simulink model "robot_joint_controlled_3_state"  (R2017b)
settings: Solver=ode8  StartTime=0.0  StopTime=2.0  FixedStep=0.00001  RelTol=1e-3
model workspace: external: MATLAB File D:\Projects\SERTS\Body\v7.0\Matlab\robot_DataFile.m (data not in the file)
values from neighbouring files (symbols this model uses):
  c_roll = 60    [best_so_far_variables.m]    (also in variables.m = 50)
  c_stance = [30,   0,    0 ... (first row only)    [best_so_far_variables.m]    (also in variables.m)
  c_swing = [50,   0,    0 ... (first row only)    [best_so_far_variables.m]    (also in variables.m = [100,   0,    0)
  c_yaw = 60    [best_so_far_variables.m]    (also in variables.m = 30)
  desired_body_height = 0.6    [best_so_far_variables.m]    (also in variables.m)
  desired_body_x_velocity = 0    [best_so_far_variables.m]    (also in variables.m)
  desired_body_y_velocity = 1    [best_so_far_variables.m]    (also in variables.m)
  desired_yaw = 0    [best_so_far_variables.m]    (also in variables.m)
  k_roll = 300    [best_so_far_variables.m]    (also in variables.m = 700)
  k_stance = [    0,    0,       0 ... (first row only)    [best_so_far_variables.m]    (also in variables.m)
  k_swing = [ 1000,     0,       0 ... (first row only)    [best_so_far_variables.m]    (also in variables.m = [02000,     0,       0)
  k_x = 0.03    [best_so_far_variables.m]    (also in variables.m)
  k_y = 0.03    [best_so_far_variables.m]    (also in variables.m)
  k_yaw = 300    [best_so_far_variables.m]    (also in variables.m)
  Left = 1    [best_so_far_variables.m]    (also in variables.m)
  LF_RH = -1    [best_so_far_variables.m]    (also in variables.m)
  lift_height = 0.05    [best_so_far_variables.m]    (also in variables.m)
  RF_LH = 1    [best_so_far_variables.m]    (also in variables.m)
  Right = -1    [best_so_far_variables.m]    (also in variables.m)
  stance_time = 0.2    [best_so_far_variables.m]    (also in variables.m)
  weight = 19    [best_so_far_variables.m]    (also in variables.m)
  width = 0.375    [best_so_far_variables.m]    (also in variables.m)
undefined symbols (not defined in the file or in its folder): smiData, X, Y, Z
libraries: sm_lib x1540, nesl_utility x44, Contact_Forces_Lib x4, simulink x4
(part 2 of 32)

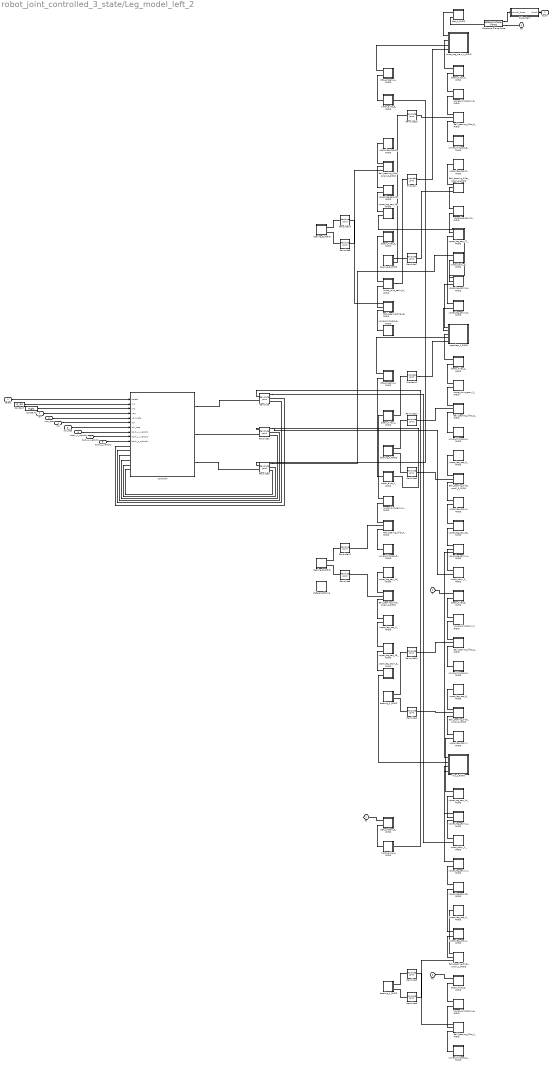
== system robot_joint_controlled_3_state/Leg_model_left_2 ==
  "select " : Inport
  "yaw " : Inport  Port=2
  yaw_rate : Inport  Port=3
  "roll " : Inport  Port=4
  roll_rate : Inport  Port=5
  body_x_velocity : Inport  Port=6
  body_y_velocity : Inport  Port=7
  body_z_velocity : Inport  Port=8
  Ball_bearing_filler_1_RIGID : Subsystem
  Ball_bearing_filler_2_RIGID : Subsystem
  Ball_bearing_filler_3_RIGID : Subsystem
  Ball_bearing_filler_4_RIGID : Subsystem
  Ball_bearing_filler_5_RIGID : Subsystem
  Ball_bearing_filler_6_RIGID : Subsystem
  Ball_bearing_filler_small_1_RIGID : Subsystem
  Ball_bearing_filler_small_2_RIGID : Subsystem
  Ball_bearing_filler_small_3_RIGID : Subsystem
  Ball_bearing_filler_small_4_RIGID : Subsystem
  Ball_bearing_filler_small_5_RIGID : Subsystem
  Ball_bearing_filler_small_6_RIGID : Subsystem
  Constant : Constant  Value=LF_RH
  Constant1 : Constant  Value=Right
  Lower_joint_cap_1_RIGID : Subsystem
  Lower_joint_cap_2_RIGID : Subsystem
  Lower_joint_cap_3_RIGID : Subsystem
  Lower_joint_cap_4_RIGID : Subsystem
  Lower_joint_cap_5_RIGID : Subsystem
  Lower_joint_cap_6_RIGID : Subsystem
  Lower_joint_casin_1_RIGID : Subsystem
  Lower_joint_casin_2_RIGID : Subsystem
  Lower_joint_casin_3_RIGID : Subsystem
  Lower_joint_casin_5_RIGID : Subsystem
  Lower_joint_casin_6_RIGID : Subsystem
  Lower_joint_casin_7_RIGID : Subsystem
  Prismatic : sm_lib/Joints/Prismatic Joint  SenseConstraintForce=off  SenseConstraintForceX=off  SenseConstraintForceY=off  SenseConstraintForceZ=off  SenseConstraintTorque=off  SenseConstraintTorqueX=off  SenseConstraintTorqueY=off  SenseConstraintTorqueZ=off  SenseTotalForce=off  SenseTotalForceX=off  SenseTotalForceY=off  SenseTotalForceZ=off  SenseTotalTorque=off  SenseTotalTorqueX=off  SenseTotalTorqueY=off  SenseTotalTorqueZ=off  CompositeWrenchDir=FollowerOnBase  CompositeWrenchFrame=BaseFrame  EquilibriumPosition=0  EquilibriumPositionUnits=m  SpringStiffness=0  SpringStiffnessUnits=N/m  DampingCoefficient=0  DampingCoefficientUnits=N/(m/s)  TorqueActuationMode=NoTorque  MotionActuationMode=ComputedMotion  SensePosition=off  SenseVelocity=off  SenseAcceleration=off  SenseTorqueForce=off  PositionTargetSpecify=on  PositionTargetPriority=Low  PositionTargetValue=smiData.PrismaticJoint(5).Pz.Pos  PositionTargetValueUnits=m  VelocityTargetSpecify=off  VelocityTargetPriority=High  VelocityTargetValue=0  VelocityTargetValueUnits=m/s
  Prismatic1 : sm_lib/Joints/Prismatic Joint  SenseConstraintForce=off  SenseConstraintForceX=off  SenseConstraintForceY=off  SenseConstraintForceZ=off  SenseConstraintTorque=off  SenseConstraintTorqueX=off  SenseConstraintTorqueY=off  SenseConstraintTorqueZ=off  SenseTotalForce=off  SenseTotalForceX=off  SenseTotalForceY=off  SenseTotalForceZ=off  SenseTotalTorque=off  SenseTotalTorqueX=off  SenseTotalTorqueY=off  SenseTotalTorqueZ=off  CompositeWrenchDir=FollowerOnBase  CompositeWrenchFrame=BaseFrame  EquilibriumPosition=0  EquilibriumPositionUnits=m  SpringStiffness=0  SpringStiffnessUnits=N/m  DampingCoefficient=0  DampingCoefficientUnits=N/(m/s)  TorqueActuationMode=NoTorque  MotionActuationMode=ComputedMotion  SensePosition=off  SenseVelocity=off  SenseAcceleration=off  SenseTorqueForce=off  PositionTargetSpecify=on  PositionTargetPriority=Low  PositionTargetValue=smiData.PrismaticJoint(6).Pz.Pos  PositionTargetValueUnits=m  VelocityTargetSpecify=off  VelocityTargetPriority=High  VelocityTargetValue=0  VelocityTargetValueUnits=m/s
  ReferenceFrame : sm_lib/Frames and Transforms/Reference Frame
  Revolute : sm_lib/Joints/Revolute Joint  SenseConstraintForce=off  SenseConstraintForceX=off  SenseConstraintForceY=off  SenseConstraintForceZ=off  SenseConstraintTorque=off  SenseConstraintTorqueX=off  SenseConstraintTorqueY=off  SenseConstraintTorqueZ=off  SenseTotalForce=off  SenseTotalForceX=off  SenseTotalForceY=off  SenseTotalForceZ=off  SenseTotalTorque=off  SenseTotalTorqueX=off  SenseTotalTorqueY=off  SenseTotalTorqueZ=off  CompositeWrenchDir=FollowerOnBase  CompositeWrenchFrame=BaseFrame  EquilibriumPosition=0  EquilibriumPositionUnits=rad  SpringStiffness=0  SpringStiffnessUnits=N*m/rad  DampingCoefficient=0  DampingCoefficientUnits=N*m/(rad/s)  TorqueActuationMode=InputTorque  MotionActuationMode=ComputedMotion  SensePosition=on  SenseVelocity=on  SenseAcceleration=off  SenseTorqueForce=off  PositionTargetSpecify=on  PositionTargetPriority=High  PositionTargetValue=0  PositionTargetValueUnits=rad  VelocityTargetSpecify=off  VelocityTargetPriority=High  VelocityTargetValue=0  VelocityTargetValueUnits=deg/s
  Revolute1 : sm_lib/Joints/Revolute Joint  SenseConstraintForce=off  SenseConstraintForceX=off  SenseConstraintForceY=off  SenseConstraintForceZ=off  SenseConstraintTorque=off  SenseConstraintTorqueX=off  SenseConstraintTorqueY=off  SenseConstraintTorqueZ=off  SenseTotalForce=off  SenseTotalForceX=off  SenseTotalForceY=off  SenseTotalForceZ=off  SenseTotalTorque=off  SenseTotalTorqueX=off  SenseTotalTorqueY=off  SenseTotalTorqueZ=off  CompositeWrenchDir=FollowerOnBase  CompositeWrenchFrame=BaseFrame  EquilibriumPosition=0  EquilibriumPositionUnits=rad  SpringStiffness=0  SpringStiffnessUnits=N*m/rad  DampingCoefficient=0  DampingCoefficientUnits=N*m/(rad/s)  TorqueActuationMode=InputTorque  MotionActuationMode=ComputedMotion  SensePosition=on  SenseVelocity=on  SenseAcceleration=off  SenseTorqueForce=off  PositionTargetSpecify=on  PositionTargetPriority=High  PositionTargetValue=0.7  PositionTargetValueUnits=rad  VelocityTargetSpecify=off  VelocityTargetPriority=High  VelocityTargetValue=0  VelocityTargetValueUnits=deg/s
  Revolute10 : sm_lib/Joints/Revolute Joint  SenseConstraintForce=off  SenseConstraintForceX=off  SenseConstraintForceY=off  SenseConstraintForceZ=off  SenseConstraintTorque=off  SenseConstraintTorqueX=off  SenseConstraintTorqueY=off  SenseConstraintTorqueZ=off  SenseTotalForce=off  SenseTotalForceX=off  SenseTotalForceY=off  SenseTotalForceZ=off  SenseTotalTorque=off  SenseTotalTorqueX=off  SenseTotalTorqueY=off  SenseTotalTorqueZ=off  CompositeWrenchDir=FollowerOnBase  CompositeWrenchFrame=BaseFrame  EquilibriumPosition=0  EquilibriumPositionUnits=rad  SpringStiffness=0  SpringStiffnessUnits=N*m/rad  DampingCoefficient=0  DampingCoefficientUnits=N*m/(rad/s)  TorqueActuationMode=NoTorque  MotionActuationMode=ComputedMotion  SensePosition=off  SenseVelocity=off  SenseAcceleration=off  SenseTorqueForce=off  PositionTargetSpecify=on  PositionTargetPriority=Low  PositionTargetValue=smiData.RevoluteJoint(41).Rz.Pos  PositionTargetValueUnits=deg  VelocityTargetSpecify=off  VelocityTargetPriority=High  VelocityTargetValue=0  VelocityTargetValueUnits=deg/s
  Revolute{3..4,11..14} (6 alike) : sm_lib/Joints/Revolute Joint  SenseConstraintForce=off  SenseConstraintForceX=off  SenseConstraintForceY=off  SenseConstraintForceZ=off  SenseConstraintTorque=off  SenseConstraintTorqueX=off  SenseConstraintTorqueY=off  SenseConstraintTorqueZ=off  SenseTotalForce=off  SenseTotalForceX=off  SenseTotalForceY=off  SenseTotalForceZ=off  SenseTotalTorque=off  SenseTotalTorqueX=off  SenseTotalTorqueY=off  SenseTotalTorqueZ=off  CompositeWrenchDir=FollowerOnBase  CompositeWrenchFrame=BaseFrame  EquilibriumPosition=0  EquilibriumPositionUnits=rad  SpringStiffness=0  SpringStiffnessUnits=N*m/rad  DampingCoefficient=0  DampingCoefficientUnits=N*m/(rad/s)  TorqueActuationMode=NoTorque  MotionActuationMode=ComputedMotion  SensePosition=off  SenseVelocity=off  SenseAcceleration=off  SenseTorqueForce=off  PositionTargetSpecify=off  PositionTargetPriority=High  PositionTargetValue=0  PositionTargetValueUnits=deg  VelocityTargetSpecify=off  VelocityTargetPriority=High  VelocityTargetValue=0  VelocityTargetValueUnits=deg/s
  Revolute2 : sm_lib/Joints/Revolute Joint  SenseConstraintForce=off  SenseConstraintForceX=off  SenseConstraintForceY=off  SenseConstraintForceZ=off  SenseConstraintTorque=off  SenseConstraintTorqueX=off  SenseConstraintTorqueY=off  SenseConstraintTorqueZ=off  SenseTotalForce=off  SenseTotalForceX=off  SenseTotalForceY=off  SenseTotalForceZ=off  SenseTotalTorque=off  SenseTotalTorqueX=off  SenseTotalTorqueY=off  SenseTotalTorqueZ=off  CompositeWrenchDir=FollowerOnBase  CompositeWrenchFrame=BaseFrame  EquilibriumPosition=0  EquilibriumPositionUnits=rad  SpringStiffness=0  SpringStiffnessUnits=N*m/rad  DampingCoefficient=0  DampingCoefficientUnits=N*m/(rad/s)  TorqueActuationMode=InputTorque  MotionActuationMode=ComputedMotion  SensePosition=on  SenseVelocity=on  SenseAcceleration=off  SenseTorqueForce=off  PositionTargetSpecify=on  PositionTargetPriority=High  PositionTargetValue=1.85  PositionTargetValueUnits=rad  VelocityTargetSpecify=off  VelocityTargetPriority=High  VelocityTargetValue=0  VelocityTargetValueUnits=deg/s
  Revolute5 : sm_lib/Joints/Revolute Joint  SenseConstraintForce=off  SenseConstraintForceX=off  SenseConstraintForceY=off  SenseConstraintForceZ=off  SenseConstraintTorque=off  SenseConstraintTorqueX=off  SenseConstraintTorqueY=off  SenseConstraintTorqueZ=off  SenseTotalForce=off  SenseTotalForceX=off  SenseTotalForceY=off  SenseTotalForceZ=off  SenseTotalTorque=off  SenseTotalTorqueX=off  SenseTotalTorqueY=off  SenseTotalTorqueZ=off  CompositeWrenchDir=FollowerOnBase  CompositeWrenchFrame=BaseFrame  EquilibriumPosition=0  EquilibriumPositionUnits=rad  SpringStiffness=0  SpringStiffnessUnits=N*m/rad  DampingCoefficient=0  DampingCoefficientUnits=N*m/(rad/s)  TorqueActuationMode=NoTorque  MotionActuationMode=ComputedMotion  SensePosition=off  SenseVelocity=off  SenseAcceleration=off  SenseTorqueForce=off  PositionTargetSpecify=on  PositionTargetPriority=Low  PositionTargetValue=smiData.RevoluteJoint(36).Rz.Pos  PositionTargetValueUnits=deg  VelocityTargetSpecify=off  VelocityTargetPriority=High  VelocityTargetValue=0  VelocityTargetValueUnits=deg/s
  Revolute6 : sm_lib/Joints/Revolute Joint  SenseConstraintForce=off  SenseConstraintForceX=off  SenseConstraintForceY=off  SenseConstraintForceZ=off  SenseConstraintTorque=off  SenseConstraintTorqueX=off  SenseConstraintTorqueY=off  SenseConstraintTorqueZ=off  SenseTotalForce=off  SenseTotalForceX=off  SenseTotalForceY=off  SenseTotalForceZ=off  SenseTotalTorque=off  SenseTotalTorqueX=off  SenseTotalTorqueY=off  SenseTotalTorqueZ=off  CompositeWrenchDir=FollowerOnBase  CompositeWrenchFrame=BaseFrame  EquilibriumPosition=0  EquilibriumPositionUnits=rad  SpringStiffness=0  SpringStiffnessUnits=N*m/rad  DampingCoefficient=0  DampingCoefficientUnits=N*m/(rad/s)  TorqueActuationMode=NoTorque  MotionActuationMode=ComputedMotion  SensePosition=off  SenseVelocity=off  SenseAcceleration=off  SenseTorqueForce=off  PositionTargetSpecify=on  PositionTargetPriority=Low  PositionTargetValue=smiData.RevoluteJoint(37).Rz.Pos  PositionTargetValueUnits=deg  VelocityTargetSpecify=off  VelocityTargetPriority=High  VelocityTargetValue=0  VelocityTargetValueUnits=deg/s
  Revolute7 : sm_lib/Joints/Revolute Joint  SenseConstraintForce=off  SenseConstraintForceX=off  SenseConstraintForceY=off  SenseConstraintForceZ=off  SenseConstraintTorque=off  SenseConstraintTorqueX=off  SenseConstraintTorqueY=off  SenseConstraintTorqueZ=off  SenseTotalForce=off  SenseTotalForceX=off  SenseTotalForceY=off  SenseTotalForceZ=off  SenseTotalTorque=off  SenseTotalTorqueX=off  SenseTotalTorqueY=off  SenseTotalTorqueZ=off  CompositeWrenchDir=FollowerOnBase  CompositeWrenchFrame=BaseFrame  EquilibriumPosition=0  EquilibriumPositionUnits=rad  SpringStiffness=0  SpringStiffnessUnits=N*m/rad  DampingCoefficient=0  DampingCoefficientUnits=N*m/(rad/s)  TorqueActuationMode=NoTorque  MotionActuationMode=ComputedMotion  SensePosition=off  SenseVelocity=off  SenseAcceleration=off  SenseTorqueForce=off  PositionTargetSpecify=on  PositionTargetPriority=Low  PositionTargetValue=smiData.RevoluteJoint(38).Rz.Pos  PositionTargetValueUnits=deg  VelocityTargetSpecify=off  VelocityTargetPriority=High  VelocityTargetValue=0  VelocityTargetValueUnits=deg/s
  Revolute8 : sm_lib/Joints/Revolute Joint  SenseConstraintForce=off  SenseConstraintForceX=off  SenseConstraintForceY=off  SenseConstraintForceZ=off  SenseConstraintTorque=off  SenseConstraintTorqueX=off  SenseConstraintTorqueY=off  SenseConstraintTorqueZ=off  SenseTotalForce=off  SenseTotalForceX=off  SenseTotalForceY=off  SenseTotalForceZ=off  SenseTotalTorque=off  SenseTotalTorqueX=off  SenseTotalTorqueY=off  SenseTotalTorqueZ=off  CompositeWrenchDir=FollowerOnBase  CompositeWrenchFrame=BaseFrame  EquilibriumPosition=0  EquilibriumPositionUnits=rad  SpringStiffness=0  SpringStiffnessUnits=N*m/rad  DampingCoefficient=0  DampingCoefficientUnits=N*m/(rad/s)  TorqueActuationMode=NoTorque  MotionActuationMode=ComputedMotion  SensePosition=off  SenseVelocity=off  SenseAcceleration=off  SenseTorqueForce=off  PositionTargetSpecify=on  PositionTargetPriority=Low  PositionTargetValue=smiData.RevoluteJoint(39).Rz.Pos  PositionTargetValueUnits=deg  VelocityTargetSpecify=off  VelocityTargetPriority=High  VelocityTargetValue=0  VelocityTargetValueUnits=deg/s
  Revolute9 : sm_lib/Joints/Revolute Joint  SenseConstraintForce=off  SenseConstraintForceX=off  SenseConstraintForceY=off  SenseConstraintForceZ=off  SenseConstraintTorque=off  SenseConstraintTorqueX=off  SenseConstraintTorqueY=off  SenseConstraintTorqueZ=off  SenseTotalForce=off  SenseTotalForceX=off  SenseTotalForceY=off  SenseTotalForceZ=off  SenseTotalTorque=off  SenseTotalTorqueX=off  SenseTotalTorqueY=off  SenseTotalTorqueZ=off  CompositeWrenchDir=FollowerOnBase  CompositeWrenchFrame=BaseFrame  EquilibriumPosition=0  EquilibriumPositionUnits=rad  SpringStiffness=0  SpringStiffnessUnits=N*m/rad  DampingCoefficient=0  DampingCoefficientUnits=N*m/(rad/s)  TorqueActuationMode=NoTorque  MotionActuationMode=ComputedMotion  SensePosition=off  SenseVelocity=off  SenseAcceleration=off  SenseTorqueForce=off  PositionTargetSpecify=on  PositionTargetPriority=Low  PositionTargetValue=smiData.RevoluteJoint(40).Rz.Pos  PositionTargetValueUnits=deg  VelocityTargetSpecify=off  VelocityTargetPriority=High  VelocityTargetValue=0  VelocityTargetValueUnits=deg/s
  SEA_system_1_RIGID : Subsystem
  SEA_system_4_RIGID : Subsystem
  SEA_system_5_RIGID : Subsystem
  Sphere to Plane Force : Contact_Forces_Lib/3D/Sphere to Plane Force  sphere_rad=0.02  plane_lenx=10  plane_leny=10  plane_depth=0.05  force_law=Linear  k_contact=38000  b_contact=38000  pen_full_damp_F=1e-4  pen_exponent=1  custom_param_1=1  custom_param_2=1  friction_law=Stick-Slip Continuous  mu_kinetic=0.8  mu_static=0.95  v_thr=0.001  vis_on=off  vis_opc_en=0  vis_len_plaBz=0.005  vis_clr=[0.9 0.2 0.2]  vis_opc=0.7
  Subsystem : Subsystem
  beam_filler_1_RIGID : Subsystem
  beam_filler_2_RIGID : Subsystem
  beam_filler_3_RIGID : Subsystem
  beam_filler_4_RIGID : Subsystem
  beam_filler_5_RIGID : Subsystem
  beam_filler_6_RIGID : Subsystem
  bearing_1_RIGID : Subsystem
  bearing_2_RIGID : Subsystem
  bearing_3_RIGID : Subsystem
  bearing_4_RIGID : Subsystem
  bearing_5_RIGID : Subsystem
  bearing_6_RIGID : Subsystem
  "controller " : Subsystem
  foot_1_RIGID : Subsystem
  hip_1_RIGID : Subsystem
  lower_leg_main_1_RIGID : Subsystem
  motor_axle_1_RIGID : Subsystem
  motor_axle_2_RIGID : Subsystem
  motor_axle_3_RIGID : Subsystem
  motor_body_1_RIGID : Subsystem
  motor_body_2_RIGID : Subsystem
  motor_body_3_RIGID : Subsystem
  upper_leg_cap_10_RIGID : Subsystem
  upper_leg_cap_11_RIGID : Subsystem
  upper_leg_cap_12_RIGID : Subsystem
  upper_leg_cap_13_RIGID : Subsystem
  upper_leg_cap_14_RIGID : Subsystem
  upper_leg_cap_15_RIGID : Subsystem
  upper_leg_cap_16_RIGID : Subsystem
  upper_leg_cap_17_RIGID : Subsystem
  upper_leg_cap_18_RIGID : Subsystem
  upper_leg_cap_1_RIGID : Subsystem
  upper_leg_cap_2_RIGID : Subsystem
  upper_leg_cap_3_RIGID : Subsystem
  upper_leg_cap_4_RIGID : Subsystem
  upper_leg_cap_5_RIGID : Subsystem
  upper_leg_cap_6_RIGID : Subsystem
  upper_leg_cap_7_RIGID : Subsystem
  upper_leg_cap_8_RIGID : Subsystem
  upper_leg_cap_9_RIGID : Subsystem
  upper_leg_casin_2_RIGID : Subsystem
  upper_leg_casin_3_RIGID : Subsystem
  upper_leg_casin_4_RIGID : Subsystem
  upper_leg_casin_5_RIGID : Subsystem
  upper_leg_casin_6_RIGID : Subsystem
  upper_leg_casin_7_RIGID : Subsystem
  upperleg_1_RIGID : Subsystem
  F3 : PMIOPort  Port=1  Side=Left
  F : PMIOPort  Port=2  Side=Left
  F1 : PMIOPort  Port=3  Side=Left
  F2 : PMIOPort  Port=4  Side=Left
  "touch " : Outport
  wires:
  Sphere to Plane Force/1 -> Subsystem/1(normal_force)
  body_z_velocity/1 -> "controller "/10(body_z_velocity)
  roll_rate/1 -> "controller "/7(roll_rate)
  body_x_velocity/1 -> "controller "/8(body_x_velocity)
  body_y_velocity/1 -> "controller "/9(body_y_velocity)
  "roll "/1 -> "controller "/6("roll ")
  "yaw "/1 -> "controller "/4("yaw ")
  Constant1/1 -> "controller "/3(In3)
  yaw_rate/1 -> "controller "/5(yaw_rate)
  "select "/1 -> "controller "/1("select ")
  Constant/1 -> "controller "/2(In2)
  Subsystem/1("touch ") -> "touch "/1
  connections:
  Ball_bearing_filler_2_RIGID/LConn3 -- Lower_joint_cap_1_RIGID/LConn1
  Ball_bearing_filler_1_RIGID/LConn3 -- Lower_joint_cap_2_RIGID/LConn1
  Ball_bearing_filler_small_5_RIGID/LConn2 -- upper_leg_cap_12_RIGID/LConn1
  upper_leg_cap_13_RIGID/LConn1 -- upper_leg_casin_7_RIGID/LConn2
  upper_leg_cap_13_RIGID/LConn2 -- upper_leg_cap_1_RIGID/LConn1
  upper_leg_cap_14_RIGID/LConn2 -- upper_leg_casin_2_RIGID/LConn2
  upper_leg_cap_14_RIGID/LConn1 -- upper_leg_cap_7_RIGID/LConn2
  upper_leg_cap_15_RIGID/LConn2 -- upper_leg_casin_4_RIGID/LConn1
  upper_leg_cap_15_RIGID/LConn1 -- upper_leg_cap_4_RIGID/LConn2
  upper_leg_cap_16_RIGID/LConn2 -- upper_leg_casin_3_RIGID/LConn1
  upper_leg_cap_16_RIGID/LConn1 -- upper_leg_cap_3_RIGID/LConn2
  upper_leg_cap_17_RIGID/LConn2 -- upper_leg_casin_5_RIGID/LConn1
  Ball_bearing_filler_4_RIGID/LConn3 -- Lower_joint_cap_3_RIGID/LConn1
  upper_leg_cap_18_RIGID/LConn2 -- upper_leg_casin_6_RIGID/LConn1
  Revolute/LConn1 -- motor_axle_1_RIGID/RConn1
  Revolute/RConn1 -- motor_body_1_RIGID/LConn2
  SEA_system_5_RIGID/LConn2 -- motor_axle_1_RIGID/LConn1
  Revolute1/LConn1 -- motor_axle_2_RIGID/RConn1
  Revolute1/RConn1 -- motor_body_2_RIGID/LConn2
  SEA_system_4_RIGID/LConn2 -- motor_axle_2_RIGID/LConn1
  Revolute2/LConn1 -- motor_axle_3_RIGID/RConn1
  Revolute2/RConn1 -- motor_body_3_RIGID/LConn1
  SEA_system_1_RIGID/LConn2 -- motor_axle_3_RIGID/LConn1
  Ball_bearing_filler_3_RIGID/LConn3 -- Lower_joint_cap_4_RIGID/LConn1
  Lower_joint_casin_5_RIGID/RConn1 -- Prismatic/LConn1
  Prismatic/RConn1 -- lower_leg_main_1_RIGID/LConn4
  Revolute3/LConn1 -- bearing_1_RIGID/RConn2
  Ball_bearing_filler_small_1_RIGID/LConn3 -- Revolute3/RConn1
  Revolute4/LConn1 -- bearing_2_RIGID/RConn2
  Ball_bearing_filler_small_2_RIGID/LConn2 -- Revolute4/RConn1
  Revolute5/LConn1 -- bearing_3_RIGID/RConn2
  Ball_bearing_filler_small_4_RIGID/LConn2 -- Revolute5/RConn1
  Revolute6/LConn1 -- bearing_4_RIGID/RConn2
  Ball_bearing_filler_small_3_RIGID/LConn2 -- Revolute6/RConn1
  Ball_bearing_filler_5_RIGID/LConn3 -- Lower_joint_cap_5_RIGID/LConn1
  Revolute7/LConn1 -- bearing_5_RIGID/RConn2
  Ball_bearing_filler_small_6_RIGID/LConn3 -- Revolute7/RConn1
  Revolute8/LConn1 -- bearing_6_RIGID/RConn2
  Ball_bearing_filler_small_5_RIGID/LConn3 -- Revolute8/RConn1
  SEA_system_4_RIGID/LConn1 -- upperleg_1_RIGID/LConn4
  SEA_system_1_RIGID/LConn1 -- lower_leg_main_1_RIGID/LConn3
  foot_1_RIGID/LConn1 -- lower_leg_main_1_RIGID/LConn1
  motor_body_1_RIGID/LConn1 -- upper_leg_casin_2_RIGID/LConn3
  motor_body_2_RIGID/LConn1 -- upper_leg_casin_4_RIGID/LConn2
  upper_leg_casin_5_RIGID/LConn2 -- upperleg_1_RIGID/LConn2
  Ball_bearing_filler_6_RIGID/LConn3 -- Lower_joint_cap_6_RIGID/LConn1
  motor_body_3_RIGID/LConn2 -- upper_leg_casin_6_RIGID/LConn2
  upper_leg_casin_6_RIGID/LConn3 -- upperleg_1_RIGID/LConn1
  Lower_joint_casin_1_RIGID/LConn1 -- beam_filler_1_RIGID/LConn1
  Prismatic1/LConn1 -- beam_filler_1_RIGID/RConn1
  Prismatic1/RConn1 -- upperleg_1_RIGID/LConn5
  Lower_joint_casin_2_RIGID/LConn1 -- beam_filler_2_RIGID/LConn2
  beam_filler_2_RIGID/LConn1 -- upperleg_1_RIGID/LConn3
  Lower_joint_casin_5_RIGID/LConn1 -- beam_filler_3_RIGID/LConn1
  Lower_joint_casin_3_RIGID/LConn1 -- beam_filler_4_RIGID/LConn2
  beam_filler_4_RIGID/LConn1 -- lower_leg_main_1_RIGID/LConn2
  Ball_bearing_filler_small_4_RIGID/LConn1 -- upper_leg_cap_10_RIGID/LConn1
  Lower_joint_casin_7_RIGID/LConn1 -- beam_filler_5_RIGID/LConn2
  Lower_joint_casin_6_RIGID/LConn1 -- beam_filler_6_RIGID/LConn2
  Ball_bearing_filler_small_1_RIGID/LConn2 -- upper_leg_cap_1_RIGID/LConn2
  Ball_bearing_filler_small_1_RIGID/LConn1 -- upper_leg_cap_2_RIGID/LConn1
  Ball_bearing_filler_small_4_RIGID/LConn3 -- upper_leg_cap_3_RIGID/LConn1
  Ball_bearing_filler_small_3_RIGID/LConn3 -- upper_leg_cap_4_RIGID/LConn1
  Ball_bearing_filler_small_6_RIGID/LConn1 -- upper_leg_cap_5_RIGID/LConn1
  Ball_bearing_filler_small_5_RIGID/LConn1 -- upper_leg_cap_6_RIGID/LConn1
  Ball_bearing_filler_small_2_RIGID/LConn3 -- upper_leg_cap_7_RIGID/LConn1
  Ball_bearing_filler_small_2_RIGID/LConn1 -- upper_leg_cap_8_RIGID/LConn1
  upper_leg_cap_11_RIGID/LConn2 -- upper_leg_cap_17_RIGID/LConn1
  Ball_bearing_filler_small_3_RIGID/LConn1 -- upper_leg_cap_9_RIGID/LConn1
  Ball_bearing_filler_1_RIGID/LConn2 -- Lower_joint_casin_6_RIGID/LConn2
  Revolute9/LConn1 -- bearing_1_RIGID/RConn1
  Ball_bearing_filler_1_RIGID/LConn1 -- Revolute9/RConn1
  Ball_bearing_filler_2_RIGID/LConn1 -- Lower_joint_casin_7_RIGID/LConn2
  Revolute10/LConn1 -- bearing_2_RIGID/RConn1
  Ball_bearing_filler_2_RIGID/LConn2 -- Revolute10/RConn1
  Ball_bearing_filler_3_RIGID/LConn1 -- Lower_joint_casin_2_RIGID/LConn2
  Revolute11/LConn1 -- bearing_4_RIGID/RConn1
  Ball_bearing_filler_3_RIGID/LConn2 -- Revolute11/RConn1
  Ball_bearing_filler_small_6_RIGID/LConn2 -- upper_leg_cap_11_RIGID/LConn1
  Ball_bearing_filler_4_RIGID/LConn1 -- Lower_joint_casin_1_RIGID/LConn2
  Revolute12/LConn1 -- bearing_3_RIGID/RConn1
  Ball_bearing_filler_4_RIGID/LConn2 -- Revolute12/RConn1
  Ball_bearing_filler_5_RIGID/LConn1 -- Lower_joint_casin_3_RIGID/LConn2
  Revolute13/LConn1 -- bearing_5_RIGID/RConn1
  Ball_bearing_filler_5_RIGID/LConn2 -- Revolute13/RConn1
  Ball_bearing_filler_6_RIGID/LConn2 -- Lower_joint_casin_5_RIGID/LConn2
  Revolute14/LConn1 -- bearing_6_RIGID/RConn1
  Ball_bearing_filler_6_RIGID/LConn1 -- Revolute14/RConn1
  hip_1_RIGID/LConn3 -- upper_leg_casin_2_RIGID/LConn1
  upper_leg_cap_12_RIGID/LConn2 -- upper_leg_cap_18_RIGID/LConn1
  hip_1_RIGID/LConn2 -- upper_leg_casin_3_RIGID/LConn2
  hip_1_RIGID/LConn1 -- upper_leg_casin_4_RIGID/LConn3
  hip_1_RIGID/LConn4 -- upper_leg_casin_7_RIGID/LConn1
  beam_filler_5_RIGID/LConn1 -- F/RConn1
  beam_filler_6_RIGID/LConn1 -- F1/RConn1
  SEA_system_5_RIGID/LConn1 -- F2/RConn1
  foot_1_RIGID/LConn2 -- Sphere to Plane Force/LConn1
  Sphere to Plane Force/RConn1 -- F3/RConn1
  "controller "/LConn3 -- Revolute1/RConn2
  "controller "/LConn6 -- Revolute2/RConn3
  "controller "/LConn5 -- Revolute2/RConn2
  "controller "/LConn4 -- Revolute1/RConn3
  "controller "/RConn3 -- Revolute2/LConn2
  "controller "/LConn2 -- Revolute/RConn3
  "controller "/RConn2 -- Revolute1/LConn2
  "controller "/LConn1 -- Revolute/RConn2
  "controller "/RConn1 -- Revolute/LConn2

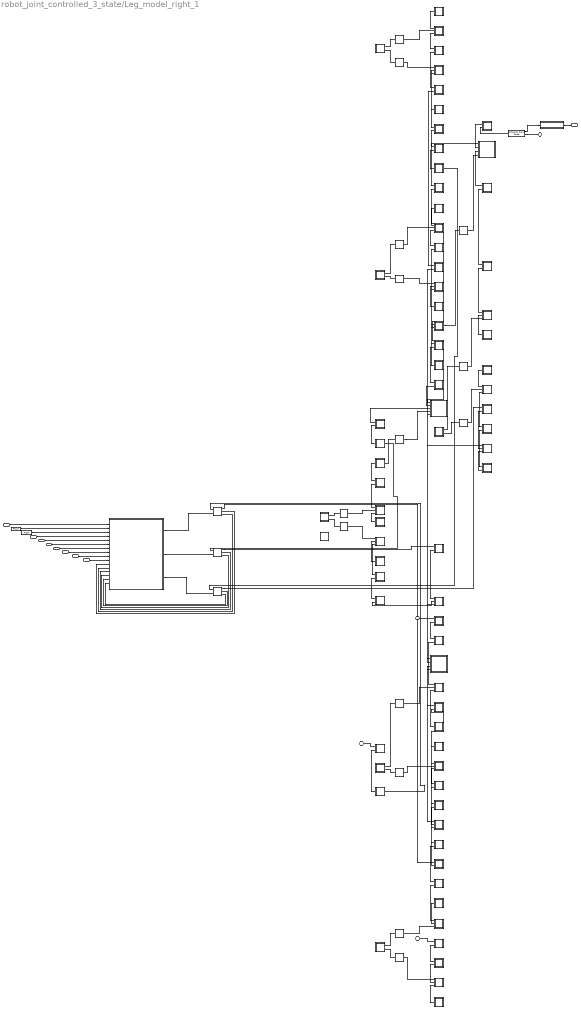
== system robot_joint_controlled_3_state/Leg_model_right_1 ==
  "select " : Inport
  "yaw " : Inport  Port=2
  yaw_rate : Inport  Port=3
  "roll " : Inport  Port=4
  roll_rate : Inport  Port=5
  body_x_velocity : Inport  Port=6
  body_y_velocity : Inport  Port=7
  body_z_velocity : Inport  Port=8
  Ball_bearing_filler_1_RIGID : Subsystem
  Ball_bearing_filler_2_RIGID : Subsystem
  Ball_bearing_filler_3_RIGID : Subsystem
  Ball_bearing_filler_4_RIGID : Subsystem
  Ball_bearing_filler_5_RIGID : Subsystem
  Ball_bearing_filler_6_RIGID : Subsystem
  Ball_bearing_filler_small_1_RIGID : Subsystem
  Ball_bearing_filler_small_2_RIGID : Subsystem
  Ball_bearing_filler_small_3_RIGID : Subsystem
  Ball_bearing_filler_small_4_RIGID : Subsystem
  Ball_bearing_filler_small_5_RIGID : Subsystem
  Ball_bearing_filler_small_6_RIGID : Subsystem
  Constant : Constant  Value=RF_LH
  Constant1 : Constant  Value=Right
  Lower_joint_cap_1_RIGID : Subsystem
  Lower_joint_cap_2_RIGID : Subsystem
  Lower_joint_cap_3_RIGID : Subsystem
  Lower_joint_cap_4_RIGID : Subsystem
  Lower_joint_cap_5_RIGID : Subsystem
  Lower_joint_cap_6_RIGID : Subsystem
  Lower_joint_casin_1_RIGID : Subsystem
  Lower_joint_casin_2_RIGID : Subsystem
  Lower_joint_casin_3_RIGID : Subsystem
  Lower_joint_casin_5_RIGID : Subsystem
  Lower_joint_casin_6_RIGID : Subsystem
  Lower_joint_casin_7_RIGID : Subsystem
  Prismatic : sm_lib/Joints/Prismatic Joint  SenseConstraintForce=off  SenseConstraintForceX=off  SenseConstraintForceY=off  SenseConstraintForceZ=off  SenseConstraintTorque=off  SenseConstraintTorqueX=off  SenseConstraintTorqueY=off  SenseConstraintTorqueZ=off  SenseTotalForce=off  SenseTotalForceX=off  SenseTotalForceY=off  SenseTotalForceZ=off  SenseTotalTorque=off  SenseTotalTorqueX=off  SenseTotalTorqueY=off  SenseTotalTorqueZ=off  CompositeWrenchDir=FollowerOnBase  CompositeWrenchFrame=BaseFrame  EquilibriumPosition=0  EquilibriumPositionUnits=m  SpringStiffness=0  SpringStiffnessUnits=N/m  DampingCoefficient=0  DampingCoefficientUnits=N/(m/s)  TorqueActuationMode=NoTorque  MotionActuationMode=ComputedMotion  SensePosition=off  SenseVelocity=off  SenseAcceleration=off  SenseTorqueForce=off  PositionTargetSpecify=on  PositionTargetPriority=Low  PositionTargetValue=smiData.PrismaticJoint(3).Pz.Pos  PositionTargetValueUnits=m  VelocityTargetSpecify=off  VelocityTargetPriority=High  VelocityTargetValue=0  VelocityTargetValueUnits=m/s
  Prismatic1 : sm_lib/Joints/Prismatic Joint  SenseConstraintForce=off  SenseConstraintForceX=off  SenseConstraintForceY=off  SenseConstraintForceZ=off  SenseConstraintTorque=off  SenseConstraintTorqueX=off  SenseConstraintTorqueY=off  SenseConstraintTorqueZ=off  SenseTotalForce=off  SenseTotalForceX=off  SenseTotalForceY=off  SenseTotalForceZ=off  SenseTotalTorque=off  SenseTotalTorqueX=off  SenseTotalTorqueY=off  SenseTotalTorqueZ=off  CompositeWrenchDir=FollowerOnBase  CompositeWrenchFrame=BaseFrame  EquilibriumPosition=0  EquilibriumPositionUnits=m  SpringStiffness=0  SpringStiffnessUnits=N/m  DampingCoefficient=0  DampingCoefficientUnits=N/(m/s)  TorqueActuationMode=NoTorque  MotionActuationMode=ComputedMotion  SensePosition=off  SenseVelocity=off  SenseAcceleration=off  SenseTorqueForce=off  PositionTargetSpecify=on  PositionTargetPriority=Low  PositionTargetValue=smiData.PrismaticJoint(4).Pz.Pos  PositionTargetValueUnits=m  VelocityTargetSpecify=off  VelocityTargetPriority=High  VelocityTargetValue=0  VelocityTargetValueUnits=m/s
  ReferenceFrame : sm_lib/Frames and Transforms/Reference Frame
  Revolute : sm_lib/Joints/Revolute Joint  SenseConstraintForce=off  SenseConstraintForceX=off  SenseConstraintForceY=off  SenseConstraintForceZ=off  SenseConstraintTorque=off  SenseConstraintTorqueX=off  SenseConstraintTorqueY=off  SenseConstraintTorqueZ=off  SenseTotalForce=off  SenseTotalForceX=off  SenseTotalForceY=off  SenseTotalForceZ=off  SenseTotalTorque=off  SenseTotalTorqueX=off  SenseTotalTorqueY=off  SenseTotalTorqueZ=off  CompositeWrenchDir=FollowerOnBase  CompositeWrenchFrame=BaseFrame  EquilibriumPosition=0  EquilibriumPositionUnits=rad  SpringStiffness=0  SpringStiffnessUnits=N*m/rad  DampingCoefficient=0  DampingCoefficientUnits=N*m/(rad/s)  TorqueActuationMode=InputTorque  MotionActuationMode=ComputedMotion  SensePosition=on  SenseVelocity=on  SenseAcceleration=off  SenseTorqueForce=off  PositionTargetSpecify=on  PositionTargetPriority=High  PositionTargetValue=0  PositionTargetValueUnits=rad  VelocityTargetSpecify=off  VelocityTargetPriority=High  VelocityTargetValue=0  VelocityTargetValueUnits=deg/s
  Revolute1 : sm_lib/Joints/Revolute Joint  SenseConstraintForce=off  SenseConstraintForceX=off  SenseConstraintForceY=off  SenseConstraintForceZ=off  SenseConstraintTorque=off  SenseConstraintTorqueX=off  SenseConstraintTorqueY=off  SenseConstraintTorqueZ=off  SenseTotalForce=off  SenseTotalForceX=off  SenseTotalForceY=off  SenseTotalForceZ=off  SenseTotalTorque=off  SenseTotalTorqueX=off  SenseTotalTorqueY=off  SenseTotalTorqueZ=off  CompositeWrenchDir=FollowerOnBase  CompositeWrenchFrame=BaseFrame  EquilibriumPosition=0  EquilibriumPositionUnits=rad  SpringStiffness=0  SpringStiffnessUnits=N*m/rad  DampingCoefficient=0  DampingCoefficientUnits=N*m/(rad/s)  TorqueActuationMode=InputTorque  MotionActuationMode=ComputedMotion  SensePosition=on  SenseVelocity=on  SenseAcceleration=off  SenseTorqueForce=off  PositionTargetSpecify=on  PositionTargetPriority=High  PositionTargetValue=0.671  PositionTargetValueUnits=rad  VelocityTargetSpecify=off  VelocityTargetPriority=High  VelocityTargetValue=0  VelocityTargetValueUnits=deg/s
  Revolute10 : sm_lib/Joints/Revolute Joint  SenseConstraintForce=off  SenseConstraintForceX=off  SenseConstraintForceY=off  SenseConstraintForceZ=off  SenseConstraintTorque=off  SenseConstraintTorqueX=off  SenseConstraintTorqueY=off  SenseConstraintTorqueZ=off  SenseTotalForce=off  SenseTotalForceX=off  SenseTotalForceY=off  SenseTotalForceZ=off  SenseTotalTorque=off  SenseTotalTorqueX=off  SenseTotalTorqueY=off  SenseTotalTorqueZ=off  CompositeWrenchDir=FollowerOnBase  CompositeWrenchFrame=BaseFrame  EquilibriumPosition=0  EquilibriumPositionUnits=rad  SpringStiffness=0  SpringStiffnessUnits=N*m/rad  DampingCoefficient=0  DampingCoefficientUnits=N*m/(rad/s)  TorqueActuationMode=NoTorque  MotionActuationMode=ComputedMotion  SensePosition=off  SenseVelocity=off  SenseAcceleration=off  SenseTorqueForce=off  PositionTargetSpecify=on  PositionTargetPriority=Low  PositionTargetValue=smiData.RevoluteJoint(26).Rz.Pos  PositionTargetValueUnits=deg  VelocityTargetSpecify=off  VelocityTargetPriority=High  VelocityTargetValue=0  VelocityTargetValueUnits=deg/s
  Revolute{3..4,11..14} (6 alike) : sm_lib/Joints/Revolute Joint  SenseConstraintForce=off  SenseConstraintForceX=off  SenseConstraintForceY=off  SenseConstraintForceZ=off  SenseConstraintTorque=off  SenseConstraintTorqueX=off  SenseConstraintTorqueY=off  SenseConstraintTorqueZ=off  SenseTotalForce=off  SenseTotalForceX=off  SenseTotalForceY=off  SenseTotalForceZ=off  SenseTotalTorque=off  SenseTotalTorqueX=off  SenseTotalTorqueY=off  SenseTotalTorqueZ=off  CompositeWrenchDir=FollowerOnBase  CompositeWrenchFrame=BaseFrame  EquilibriumPosition=0  EquilibriumPositionUnits=rad  SpringStiffness=0  SpringStiffnessUnits=N*m/rad  DampingCoefficient=0  DampingCoefficientUnits=N*m/(rad/s)  TorqueActuationMode=NoTorque  MotionActuationMode=ComputedMotion  SensePosition=off  SenseVelocity=off  SenseAcceleration=off  SenseTorqueForce=off  PositionTargetSpecify=off  PositionTargetPriority=High  PositionTargetValue=0  PositionTargetValueUnits=deg  VelocityTargetSpecify=off  VelocityTargetPriority=High  VelocityTargetValue=0  VelocityTargetValueUnits=deg/s
  Revolute2 : sm_lib/Joints/Revolute Joint  SenseConstraintForce=off  SenseConstraintForceX=off  SenseConstraintForceY=off  SenseConstraintForceZ=off  SenseConstraintTorque=off  SenseConstraintTorqueX=off  SenseConstraintTorqueY=off  SenseConstraintTorqueZ=off  SenseTotalForce=off  SenseTotalForceX=off  SenseTotalForceY=off  SenseTotalForceZ=off  SenseTotalTorque=off  SenseTotalTorqueX=off  SenseTotalTorqueY=off  SenseTotalTorqueZ=off  CompositeWrenchDir=FollowerOnBase  CompositeWrenchFrame=BaseFrame  EquilibriumPosition=0  EquilibriumPositionUnits=rad  SpringStiffness=0  SpringStiffnessUnits=N*m/rad  DampingCoefficient=0  DampingCoefficientUnits=N*m/(rad/s)  TorqueActuationMode=InputTorque  MotionActuationMode=ComputedMotion  SensePosition=on  SenseVelocity=on  SenseAcceleration=off  SenseTorqueForce=off  PositionTargetSpecify=on  PositionTargetPriority=Low  PositionTargetValue=4.360  PositionTargetValueUnits=rad  VelocityTargetSpecify=off  VelocityTargetPriority=High  VelocityTargetValue=0  VelocityTargetValueUnits=deg/s
  Revolute5 : sm_lib/Joints/Revolute Joint  SenseConstraintForce=off  SenseConstraintForceX=off  SenseConstraintForceY=off  SenseConstraintForceZ=off  SenseConstraintTorque=off  SenseConstraintTorqueX=off  SenseConstraintTorqueY=off  SenseConstraintTorqueZ=off  SenseTotalForce=off  SenseTotalForceX=off  SenseTotalForceY=off  SenseTotalForceZ=off  SenseTotalTorque=off  SenseTotalTorqueX=off  SenseTotalTorqueY=off  SenseTotalTorqueZ=off  CompositeWrenchDir=FollowerOnBase  CompositeWrenchFrame=BaseFrame  EquilibriumPosition=0  EquilibriumPositionUnits=rad  SpringStiffness=0  SpringStiffnessUnits=N*m/rad  DampingCoefficient=0  DampingCoefficientUnits=N*m/(rad/s)  TorqueActuationMode=NoTorque  MotionActuationMode=ComputedMotion  SensePosition=off  SenseVelocity=off  SenseAcceleration=off  SenseTorqueForce=off  PositionTargetSpecify=on  PositionTargetPriority=Low  PositionTargetValue=smiData.RevoluteJoint(21).Rz.Pos  PositionTargetValueUnits=deg  VelocityTargetSpecify=off  VelocityTargetPriority=High  VelocityTargetValue=0  VelocityTargetValueUnits=deg/s
  Revolute6 : sm_lib/Joints/Revolute Joint  SenseConstraintForce=off  SenseConstraintForceX=off  SenseConstraintForceY=off  SenseConstraintForceZ=off  SenseConstraintTorque=off  SenseConstraintTorqueX=off  SenseConstraintTorqueY=off  SenseConstraintTorqueZ=off  SenseTotalForce=off  SenseTotalForceX=off  SenseTotalForceY=off  SenseTotalForceZ=off  SenseTotalTorque=off  SenseTotalTorqueX=off  SenseTotalTorqueY=off  SenseTotalTorqueZ=off  CompositeWrenchDir=FollowerOnBase  CompositeWrenchFrame=BaseFrame  EquilibriumPosition=0  EquilibriumPositionUnits=rad  SpringStiffness=0  SpringStiffnessUnits=N*m/rad  DampingCoefficient=0  DampingCoefficientUnits=N*m/(rad/s)  TorqueActuationMode=NoTorque  MotionActuationMode=ComputedMotion  SensePosition=off  SenseVelocity=off  SenseAcceleration=off  SenseTorqueForce=off  PositionTargetSpecify=on  PositionTargetPriority=Low  PositionTargetValue=smiData.RevoluteJoint(22).Rz.Pos  PositionTargetValueUnits=deg  VelocityTargetSpecify=off  VelocityTargetPriority=High  VelocityTargetValue=0  VelocityTargetValueUnits=deg/s
  Revolute7 : sm_lib/Joints/Revolute Joint  SenseConstraintForce=off  SenseConstraintForceX=off  SenseConstraintForceY=off  SenseConstraintForceZ=off  SenseConstraintTorque=off  SenseConstraintTorqueX=off  SenseConstraintTorqueY=off  SenseConstraintTorqueZ=off  SenseTotalForce=off  SenseTotalForceX=off  SenseTotalForceY=off  SenseTotalForceZ=off  SenseTotalTorque=off  SenseTotalTorqueX=off  SenseTotalTorqueY=off  SenseTotalTorqueZ=off  CompositeWrenchDir=FollowerOnBase  CompositeWrenchFrame=BaseFrame  EquilibriumPosition=0  EquilibriumPositionUnits=rad  SpringStiffness=0  SpringStiffnessUnits=N*m/rad  DampingCoefficient=0  DampingCoefficientUnits=N*m/(rad/s)  TorqueActuationMode=NoTorque  MotionActuationMode=ComputedMotion  SensePosition=off  SenseVelocity=off  SenseAcceleration=off  SenseTorqueForce=off  PositionTargetSpecify=on  PositionTargetPriority=Low  PositionTargetValue=smiData.RevoluteJoint(23).Rz.Pos  PositionTargetValueUnits=deg  VelocityTargetSpecify=off  VelocityTargetPriority=High  VelocityTargetValue=0  VelocityTargetValueUnits=deg/s
  Revolute8 : sm_lib/Joints/Revolute Joint  SenseConstraintForce=off  SenseConstraintForceX=off  SenseConstraintForceY=off  SenseConstraintForceZ=off  SenseConstraintTorque=off  SenseConstraintTorqueX=off  SenseConstraintTorqueY=off  SenseConstraintTorqueZ=off  SenseTotalForce=off  SenseTotalForceX=off  SenseTotalForceY=off  SenseTotalForceZ=off  SenseTotalTorque=off  SenseTotalTorqueX=off  SenseTotalTorqueY=off  SenseTotalTorqueZ=off  CompositeWrenchDir=FollowerOnBase  CompositeWrenchFrame=BaseFrame  EquilibriumPosition=0  EquilibriumPositionUnits=rad  SpringStiffness=0  SpringStiffnessUnits=N*m/rad  DampingCoefficient=0  DampingCoefficientUnits=N*m/(rad/s)  TorqueActuationMode=NoTorque  MotionActuationMode=ComputedMotion  SensePosition=off  SenseVelocity=off  SenseAcceleration=off  SenseTorqueForce=off  PositionTargetSpecify=on  PositionTargetPriority=Low  PositionTargetValue=smiData.RevoluteJoint(24).Rz.Pos  PositionTargetValueUnits=deg  VelocityTargetSpecify=off  VelocityTargetPriority=High  VelocityTargetValue=0  VelocityTargetValueUnits=deg/s
  Revolute9 : sm_lib/Joints/Revolute Joint  SenseConstraintForce=off  SenseConstraintForceX=off  SenseConstraintForceY=off  SenseConstraintForceZ=off  SenseConstraintTorque=off  SenseConstraintTorqueX=off  SenseConstraintTorqueY=off  SenseConstraintTorqueZ=off  SenseTotalForce=off  SenseTotalForceX=off  SenseTotalForceY=off  SenseTotalForceZ=off  SenseTotalTorque=off  SenseTotalTorqueX=off  SenseTotalTorqueY=off  SenseTotalTorqueZ=off  CompositeWrenchDir=FollowerOnBase  CompositeWrenchFrame=BaseFrame  EquilibriumPosition=0  EquilibriumPositionUnits=rad  SpringStiffness=0  SpringStiffnessUnits=N*m/rad  DampingCoefficient=0  DampingCoefficientUnits=N*m/(rad/s)  TorqueActuationMode=NoTorque  MotionActuationMode=ComputedMotion  SensePosition=off  SenseVelocity=off  SenseAcceleration=off  SenseTorqueForce=off  PositionTargetSpecify=on  PositionTargetPriority=Low  PositionTargetValue=smiData.RevoluteJoint(25).Rz.Pos  PositionTargetValueUnits=deg  VelocityTargetSpecify=off  VelocityTargetPriority=High  VelocityTargetValue=0  VelocityTargetValueUnits=deg/s
  SEA_system_1_RIGID : Subsystem
  SEA_system_4_RIGID : Subsystem
  SEA_system_5_RIGID : Subsystem
  Sphere to Plane Force : Contact_Forces_Lib/3D/Sphere to Plane Force  sphere_rad=0.02  plane_lenx=10  plane_leny=10  plane_depth=0.05  force_law=Linear  k_contact=38000  b_contact=38000  pen_full_damp_F=1e-4  pen_exponent=1  custom_param_1=1  custom_param_2=1  friction_law=Stick-Slip Continuous  mu_kinetic=0.8  mu_static=0.95  v_thr=0.001  vis_on=off  vis_opc_en=0  vis_len_plaBz=0.005  vis_clr=[0.9 0.2 0.2]  vis_opc=0.7
  Subsystem : Subsystem
  beam_filler_1_RIGID : Subsystem
  beam_filler_2_RIGID : Subsystem
  beam_filler_3_RIGID : Subsystem
  beam_filler_4_RIGID : Subsystem
  beam_filler_5_RIGID : Subsystem
  beam_filler_6_RIGID : Subsystem
  bearing_1_RIGID : Subsystem
  bearing_2_RIGID : Subsystem
  bearing_3_RIGID : Subsystem
  bearing_4_RIGID : Subsystem
  bearing_5_RIGID : Subsystem
  bearing_6_RIGID : Subsystem
  "controller " : Subsystem
  foot_1_RIGID : Subsystem
  hip_1_RIGID : Subsystem
  lower_leg_main_1_RIGID : Subsystem
  motor_axle_1_RIGID : Subsystem
  motor_axle_2_RIGID : Subsystem
  motor_axle_3_RIGID : Subsystem
  motor_body_1_RIGID : Subsystem
  motor_body_2_RIGID : Subsystem
  motor_body_3_RIGID : Subsystem
  upper_leg_cap_10_RIGID : Subsystem
  upper_leg_cap_11_RIGID : Subsystem
  upper_leg_cap_12_RIGID : Subsystem
  upper_leg_cap_13_RIGID : Subsystem
  upper_leg_cap_14_RIGID : Subsystem
  upper_leg_cap_15_RIGID : Subsystem
  upper_leg_cap_16_RIGID : Subsystem
  upper_leg_cap_17_RIGID : Subsystem
  upper_leg_cap_18_RIGID : Subsystem
  upper_leg_cap_1_RIGID : Subsystem
  upper_leg_cap_2_RIGID : Subsystem
  upper_leg_cap_3_RIGID : Subsystem
  upper_leg_cap_4_RIGID : Subsystem
  upper_leg_cap_5_RIGID : Subsystem
  upper_leg_cap_6_RIGID : Subsystem
  upper_leg_cap_7_RIGID : Subsystem
  upper_leg_cap_8_RIGID : Subsystem
  upper_leg_cap_9_RIGID : Subsystem
  upper_leg_casin_2_RIGID : Subsystem
  upper_leg_casin_3_RIGID : Subsystem
  upper_leg_casin_4_RIGID : Subsystem
  upper_leg_casin_5_RIGID : Subsystem
  upper_leg_casin_6_RIGID : Subsystem
  upper_leg_casin_7_RIGID : Subsystem
  upperleg_1_RIGID : Subsystem
  F3 : PMIOPort  Port=1  Side=Left
  F : PMIOPort  Port=2  Side=Left
  F1 : PMIOPort  Port=3  Side=Left
  F2 : PMIOPort  Port=4  Side=Left
  "touch " : Outport
  wires:
  Sphere to Plane Force/1 -> Subsystem/1(normal_force)
  body_z_velocity/1 -> "controller "/10(body_z_velocity)
  roll_rate/1 -> "controller "/7(roll_rate)
  body_x_velocity/1 -> "controller "/8(body_x_velocity)
  body_y_velocity/1 -> "controller "/9(body_y_velocity)
  "roll "/1 -> "controller "/6("roll ")
  "yaw "/1 -> "controller "/4("yaw ")
  Constant1/1 -> "controller "/3(In3)
  yaw_rate/1 -> "controller "/5(yaw_rate)
  "select "/1 -> "controller "/1("select ")
  Constant/1 -> "controller "/2(In2)
  Subsystem/1("touch ") -> "touch "/1
  connections:
  Ball_bearing_filler_2_RIGID/LConn3 -- Lower_joint_cap_1_RIGID/LConn1
  Ball_bearing_filler_1_RIGID/LConn3 -- Lower_joint_cap_2_RIGID/LConn1
  Ball_bearing_filler_small_5_RIGID/LConn3 -- upper_leg_cap_12_RIGID/LConn1
  upper_leg_cap_13_RIGID/LConn1 -- upper_leg_casin_7_RIGID/LConn2
  upper_leg_cap_13_RIGID/LConn2 -- upper_leg_cap_1_RIGID/LConn1
  upper_leg_cap_14_RIGID/LConn2 -- upper_leg_casin_2_RIGID/LConn2
  upper_leg_cap_14_RIGID/LConn1 -- upper_leg_cap_7_RIGID/LConn2
  upper_leg_cap_15_RIGID/LConn2 -- upper_leg_casin_4_RIGID/LConn1
  upper_leg_cap_15_RIGID/LConn1 -- upper_leg_cap_4_RIGID/LConn2
  upper_leg_cap_16_RIGID/LConn2 -- upper_leg_casin_3_RIGID/LConn2
  upper_leg_cap_16_RIGID/LConn1 -- upper_leg_cap_3_RIGID/LConn2
  upper_leg_cap_17_RIGID/LConn2 -- upper_leg_casin_5_RIGID/LConn3
  Ball_bearing_filler_4_RIGID/LConn3 -- Lower_joint_cap_3_RIGID/LConn1
  upper_leg_cap_18_RIGID/LConn2 -- upper_leg_casin_6_RIGID/LConn1
  Revolute/LConn1 -- motor_axle_1_RIGID/RConn1
  Revolute/RConn1 -- motor_body_1_RIGID/LConn1
  SEA_system_5_RIGID/LConn2 -- motor_axle_1_RIGID/LConn1
  Revolute1/LConn1 -- motor_axle_2_RIGID/RConn1
  Revolute1/RConn1 -- motor_body_2_RIGID/LConn1
  SEA_system_4_RIGID/LConn2 -- motor_axle_2_RIGID/LConn1
  Revolute2/LConn1 -- motor_axle_3_RIGID/RConn1
  Revolute2/RConn1 -- motor_body_3_RIGID/LConn1
  SEA_system_1_RIGID/LConn2 -- motor_axle_3_RIGID/LConn1
  Ball_bearing_filler_3_RIGID/LConn2 -- Lower_joint_cap_4_RIGID/LConn1
  Lower_joint_casin_5_RIGID/RConn1 -- Prismatic/LConn1
  Prismatic/RConn1 -- lower_leg_main_1_RIGID/LConn4
  Revolute3/LConn1 -- bearing_1_RIGID/RConn1
  Ball_bearing_filler_small_1_RIGID/LConn3 -- Revolute3/RConn1
  Revolute4/LConn1 -- bearing_2_RIGID/RConn2
  Ball_bearing_filler_small_2_RIGID/LConn2 -- Revolute4/RConn1
  Revolute5/LConn1 -- bearing_3_RIGID/RConn2
  Ball_bearing_filler_small_4_RIGID/LConn1 -- Revolute5/RConn1
  Revolute6/LConn1 -- bearing_4_RIGID/RConn1
  Ball_bearing_filler_small_3_RIGID/LConn2 -- Revolute6/RConn1
  Ball_bearing_filler_5_RIGID/LConn2 -- Lower_joint_cap_5_RIGID/LConn1
  Revolute7/LConn1 -- bearing_5_RIGID/RConn2
  Ball_bearing_filler_small_6_RIGID/LConn2 -- Revolute7/RConn1
  Revolute8/LConn1 -- bearing_6_RIGID/RConn1
  Ball_bearing_filler_small_5_RIGID/LConn2 -- Revolute8/RConn1
  SEA_system_4_RIGID/LConn1 -- upperleg_1_RIGID/LConn3
  SEA_system_1_RIGID/LConn1 -- lower_leg_main_1_RIGID/LConn2
  foot_1_RIGID/LConn1 -- lower_leg_main_1_RIGID/LConn1
  motor_body_1_RIGID/LConn2 -- upper_leg_casin_2_RIGID/LConn3
  motor_body_2_RIGID/LConn2 -- upper_leg_casin_3_RIGID/LConn1
  motor_body_3_RIGID/LConn2 -- upper_leg_casin_5_RIGID/LConn2
  Ball_bearing_filler_6_RIGID/LConn2 -- Lower_joint_cap_6_RIGID/LConn1
  upper_leg_casin_5_RIGID/LConn1 -- upperleg_1_RIGID/LConn5
  upper_leg_casin_6_RIGID/LConn2 -- upperleg_1_RIGID/LConn2
  Lower_joint_casin_1_RIGID/LConn1 -- beam_filler_1_RIGID/LConn1
  Prismatic1/LConn1 -- beam_filler_1_RIGID/RConn1
  Prismatic1/RConn1 -- upperleg_1_RIGID/LConn4
  Lower_joint_casin_2_RIGID/LConn2 -- beam_filler_2_RIGID/LConn1
  beam_filler_2_RIGID/LConn2 -- upperleg_1_RIGID/LConn1
  Lower_joint_casin_5_RIGID/LConn2 -- beam_filler_3_RIGID/LConn1
  Lower_joint_casin_3_RIGID/LConn1 -- beam_filler_4_RIGID/LConn2
  beam_filler_4_RIGID/LConn1 -- lower_leg_main_1_RIGID/LConn3
  Ball_bearing_filler_small_4_RIGID/LConn2 -- upper_leg_cap_10_RIGID/LConn1
  Lower_joint_casin_7_RIGID/LConn1 -- beam_filler_5_RIGID/LConn2
  Lower_joint_casin_6_RIGID/LConn1 -- beam_filler_6_RIGID/LConn2
  Ball_bearing_filler_small_1_RIGID/LConn1 -- upper_leg_cap_1_RIGID/LConn2
  Ball_bearing_filler_small_1_RIGID/LConn2 -- upper_leg_cap_2_RIGID/LConn1
  Ball_bearing_filler_small_4_RIGID/LConn3 -- upper_leg_cap_3_RIGID/LConn1
  Ball_bearing_filler_small_3_RIGID/LConn3 -- upper_leg_cap_4_RIGID/LConn1
  Ball_bearing_filler_small_6_RIGID/LConn1 -- upper_leg_cap_5_RIGID/LConn1
  Ball_bearing_filler_small_5_RIGID/LConn1 -- upper_leg_cap_6_RIGID/LConn1
  Ball_bearing_filler_small_2_RIGID/LConn3 -- upper_leg_cap_7_RIGID/LConn1
  Ball_bearing_filler_small_2_RIGID/LConn1 -- upper_leg_cap_8_RIGID/LConn1
  upper_leg_cap_11_RIGID/LConn2 -- upper_leg_cap_17_RIGID/LConn1
  Ball_bearing_filler_small_3_RIGID/LConn1 -- upper_leg_cap_9_RIGID/LConn1
  Ball_bearing_filler_1_RIGID/LConn2 -- Lower_joint_casin_6_RIGID/LConn2
  Revolute9/LConn1 -- bearing_1_RIGID/RConn2
  Ball_bearing_filler_1_RIGID/LConn1 -- Revolute9/RConn1
  Ball_bearing_filler_2_RIGID/LConn1 -- Lower_joint_casin_7_RIGID/LConn2
  Revolute10/LConn1 -- bearing_2_RIGID/RConn1
  Ball_bearing_filler_2_RIGID/LConn2 -- Revolute10/RConn1
  Ball_bearing_filler_3_RIGID/LConn3 -- Lower_joint_casin_2_RIGID/LConn1
  Revolute11/LConn1 -- bearing_4_RIGID/RConn2
  Ball_bearing_filler_3_RIGID/LConn1 -- Revolute11/RConn1
  Ball_bearing_filler_small_6_RIGID/LConn3 -- upper_leg_cap_11_RIGID/LConn1
  Ball_bearing_filler_4_RIGID/LConn1 -- Lower_joint_casin_1_RIGID/LConn2
  Revolute12/LConn1 -- bearing_3_RIGID/RConn1
  Ball_bearing_filler_4_RIGID/LConn2 -- Revolute12/RConn1
  Ball_bearing_filler_5_RIGID/LConn1 -- Lower_joint_casin_3_RIGID/LConn2
  Revolute13/LConn1 -- bearing_5_RIGID/RConn1
  Ball_bearing_filler_5_RIGID/LConn3 -- Revolute13/RConn1
  Ball_bearing_filler_6_RIGID/LConn3 -- Lower_joint_casin_5_RIGID/LConn1
  Revolute14/LConn1 -- bearing_6_RIGID/RConn2
  Ball_bearing_filler_6_RIGID/LConn1 -- Revolute14/RConn1
  hip_1_RIGID/LConn4 -- upper_leg_casin_2_RIGID/LConn1
  upper_leg_cap_12_RIGID/LConn2 -- upper_leg_cap_18_RIGID/LConn1
  hip_1_RIGID/LConn2 -- upper_leg_casin_3_RIGID/LConn3
  hip_1_RIGID/LConn1 -- upper_leg_casin_4_RIGID/LConn2
  hip_1_RIGID/LConn3 -- upper_leg_casin_7_RIGID/LConn1
  SEA_system_5_RIGID/LConn1 -- F/RConn1
  beam_filler_5_RIGID/LConn1 -- F1/RConn1
  beam_filler_6_RIGID/LConn1 -- F2/RConn1
  foot_1_RIGID/LConn2 -- Sphere to Plane Force/LConn1
  Sphere to Plane Force/RConn1 -- F3/RConn1
  "controller "/LConn3 -- Revolute1/RConn2
  "controller "/LConn6 -- Revolute2/RConn3
  "controller "/LConn5 -- Revolute2/RConn2
  "controller "/LConn4 -- Revolute1/RConn3
  "controller "/RConn3 -- Revolute2/LConn2
  "controller "/LConn2 -- Revolute/RConn3
  "controller "/RConn2 -- Revolute1/LConn2
  "controller "/LConn1 -- Revolute/RConn2
  "controller "/RConn1 -- Revolute/LConn2
